simulink model "lab63"  (Simulink 8.0)
settings: Solver=ode45  StartTime=0.0  StopTime=10.0  RelTol=1e-3
libraries: commdigbbndpm3 x3, commchan3 x2, commrandsrc2 x1, commsink2 x1
settings Model: Creator=Dimav  LastModifiedBy=Dimav

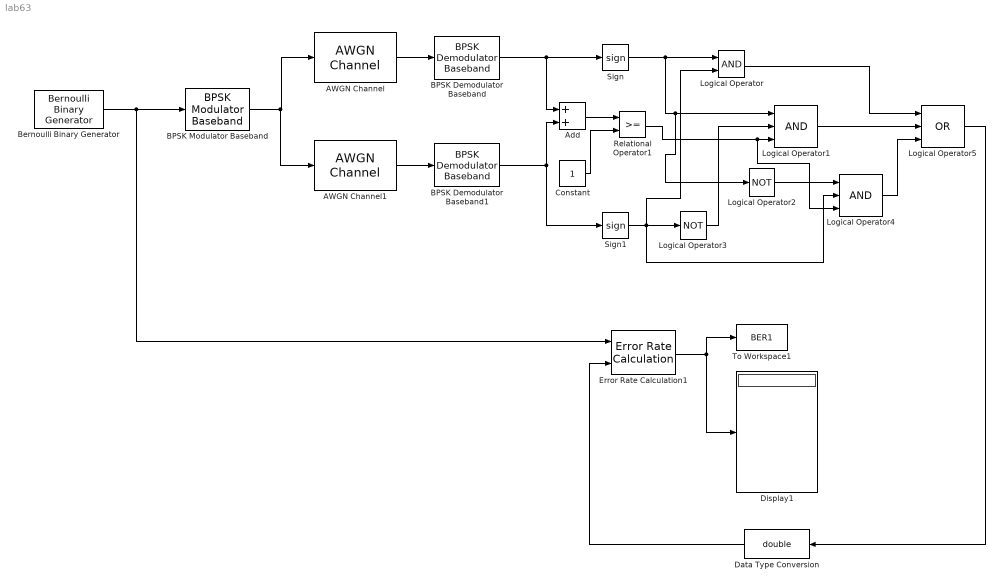
== system lab63 ==
  AWGN Channel : commchan3/AWGN Channel  InputProcessing=Columns as channels (frame based)  seed=67  noiseMode="Signal to noise ratio  (Eb/No)"  EbNodB=3  EsNodB=10  SNRdB=10  bitsPerSym=1  Ps=1  Tsym=1/1200  variance=1
  AWGN Channel1 : commchan3/AWGN Channel  InputProcessing=Columns as channels (frame based)  seed=67  noiseMode="Signal to noise ratio  (Eb/No)"  EbNodB=10  EsNodB=10  SNRdB=10  bitsPerSym=1  Ps=1  Tsym=1/1200  variance=1
  Add : Sum
  BPSK Demodulator Baseband : commdigbbndpm3/BPSK Demodulator Baseband  Ph=0  DecType=Hard decision  VarSource=Dialog  Variance=1  outDtype=Inherit via internal rule  derotateFactorWordLen=16
  BPSK Demodulator Baseband1 : commdigbbndpm3/BPSK Demodulator Baseband  Ph=0  DecType=Hard decision  VarSource=Dialog  Variance=1  outDtype=Inherit via internal rule  derotateFactorWordLen=16
  BPSK Modulator Baseband : commdigbbndpm3/BPSK Modulator Baseband  Ph=0  outDtype=double  outWordLen=16  outUDDataType=sfix(16)  outFracLenMode=Best precision  outFracLen=15
  Bernoulli Binary Generator : commrandsrc2/Bernoulli Binary Generator  P=0.5  seed=61  Ts=1/1200  frameBased=on  sampPerFrame=1  orient=off  outDataType=double
  Constant : Constant
  Data Type Conversion : DataTypeConversion  OutDataTypeStr=double
  Display1 : Display
  Error Rate Calculation1 : commsink2/Error Rate Calculation  N=0  st_delay=0  cp_mode=Entire frame  subframe=[]  PMode=Port  WsName=ErrorVec  RsMode2=off  stop=off  numErr=100  maxBits=1e6
  Logical Operator : Logic  AllPortsSameDT=off  OutDataTypeStr=boolean
  Logical Operator1 : Logic  Inputs=3  AllPortsSameDT=off  OutDataTypeStr=boolean
  Logical Operator2 : Logic  Operator=NOT  AllPortsSameDT=off  OutDataTypeStr=boolean
  Logical Operator3 : Logic  Operator=NOT  AllPortsSameDT=off  OutDataTypeStr=boolean
  Logical Operator4 : Logic  Inputs=3  AllPortsSameDT=off  OutDataTypeStr=boolean
  Logical Operator5 : Logic  Operator=OR  Inputs=3  AllPortsSameDT=off  OutDataTypeStr=boolean
  Relational Operator1 : RelationalOperator  OutDataTypeStr=boolean
  Sign : Signum
  Sign1 : Signum
  To Workspace1 : ToWorkspace  VariableName=BER1  SampleTime=-1  SaveFormat=Timeseries
  wires:
  Bernoulli Binary Generator/1 -> Error Rate Calculation1/1, BPSK Modulator Baseband/1
  BPSK Modulator Baseband/1 -> AWGN Channel1/1, AWGN Channel/1
  BPSK Demodulator Baseband/1 -> Sign/1, Add/1
  AWGN Channel1/1 -> BPSK Demodulator Baseband1/1
  AWGN Channel/1 -> BPSK Demodulator Baseband/1
  Error Rate Calculation1/1 -> To Workspace1/1, Display1/1
  Sign/1 -> Logical Operator1/1, Logical Operator2/1, Logical Operator/1
  Add/1 -> Relational Operator1/1
  Constant/1 -> Relational Operator1/2
  BPSK Demodulator Baseband1/1 -> Sign1/1, Add/2
  Sign1/1 -> Logical Operator4/2, Logical Operator/2, Logical Operator3/1
  Logical Operator3/1 -> Logical Operator1/2
  Relational Operator1/1 -> Logical Operator4/3, Logical Operator1/3
  Logical Operator2/1 -> Logical Operator4/1
  Logical Operator/1 -> Logical Operator5/1
  Logical Operator1/1 -> Logical Operator5/2
  Logical Operator4/1 -> Logical Operator5/3
  Logical Operator5/1 -> Data Type Conversion/1
  Data Type Conversion/1 -> Error Rate Calculation1/2
